simulink model "sigRecPlay"  (Simulink 6.1)
settings: Solver=FixedStepDiscrete  StartTime=0.0  StopTime=100  FixedStep=0.1  RelTol=1e-3
libraries: simulink x2
settings Model: LastModifiedBy=murahasi
settings DebuggingCC: SolverPrmCheckMsg=warning

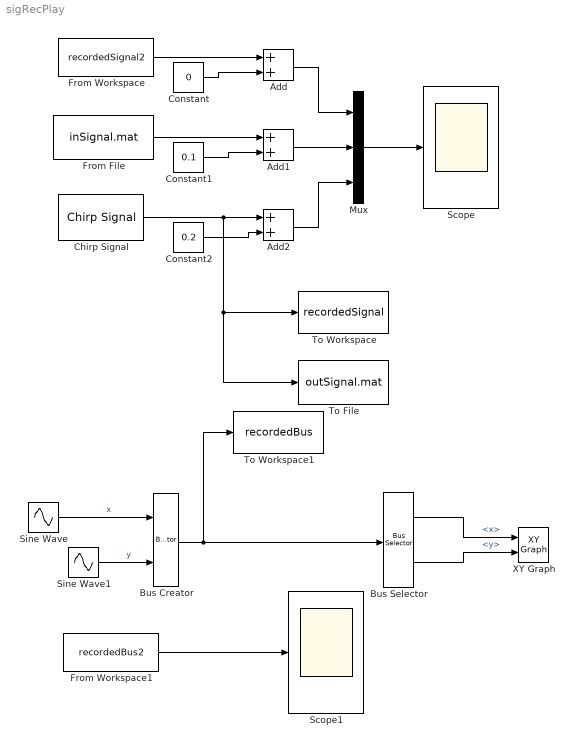
== system sigRecPlay ==
  Add : Sum  OutScaling=2^-10
  Add1 : Sum  OutScaling=2^-10
  Add2 : Sum  OutScaling=2^-10
  Bus Creator : BusCreator  DialogController=Simulink.DDGSource_Bus  Inputs=2
  Bus Selector : BusSelector  DialogController=Simulink.DDGSource_Bus  OutputSignals=x,y
  Chirp Signal : simulink/Sources/Chirp Signal  f1=0.1  T=100  f2=1
  Constant : Constant  Value=0
  Constant1 : Constant  Value=0.1
  Constant2 : Constant  Value=0.2
  From Workspace : FromWorkspace  VariableName=recordedSignal2  SampleTime=0.1  Interpolate=off  OutputAfterFinalValue=Holding final value
  From Workspace1 : FromWorkspace  VariableName=recordedBus2  SampleTime=0.1  Interpolate=off  OutputAfterFinalValue=Holding final value
  From File : FromFile  FileName=inSignal.mat  SampleTime=0.1
  Mux : Mux  Inputs=3
  Scope : Scope
  Scope1 : Scope
  Sine Wave : Sin  SineType=Sample based  Samples=36  SampleTime=0.1  Offset=9
  Sine Wave1 : Sin  SineType=Sample based  Samples=36  SampleTime=0.1
  To File : ToFile  Filename=outSignal.mat
  To Workspace : ToWorkspace  VariableName=recordedSignal  SampleTime=0.1  SaveFormat=Structure
  To Workspace1 : ToWorkspace  VariableName=recordedBus  SampleTime=0.1  SaveFormat=Structure
  XY Graph : simulink/Sinks/XY Graph  xmin=-1  xmax=1  ymin=-1  ymax=1  st=-1
  wires:
  Chirp Signal/1 -> To Workspace/1, To File/1, Add2/1
  From Workspace/1 -> Add/1
  From File/1 -> Add1/1
  Constant/1 -> Add/2
  Constant1/1 -> Add1/2
  Constant2/1 -> Add2/2
  Add/1 -> Mux/1
  Add1/1 -> Mux/2
  Add2/1 -> Mux/3
  Mux/1 -> Scope/1
  Bus Creator/1 -> To Workspace1/1, Bus Selector/1
  Bus Selector/1 -> XY Graph/1  "<x>"
  Bus Selector/2 -> XY Graph/2  "<y>"
  Sine Wave/1 -> Bus Creator/1  "x"
  Sine Wave1/1 -> Bus Creator/2  "y"
  From Workspace1/1 -> Scope1/1
